simulink model "Standard"  (R2015a)
settings: Solver=ode45  StartTime=0.0  StopTime=300  RelTol=1e-3
undefined symbols (not defined in the file): A, B_cont, B_dist, dt, SegNum
settings Model: Creator=Nick  LastModifiedBy=Nick

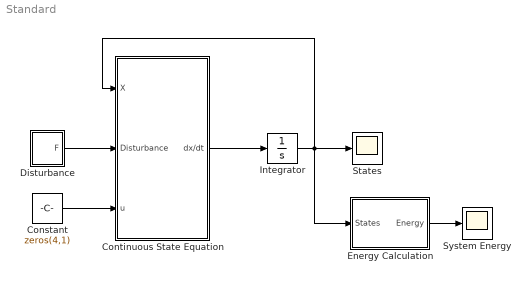
== system Standard ==
  Constant : Constant  Value=zeros(4,1)
  Continuous State Equation : Subsystem
  Disturbance : Subsystem
  Energy Calculation : Subsystem
  Integrator : Integrator
  States : Scope
      settings: SaveName=StandardStates
  System Energy : Scope
      settings: YMin=-5.65455e-27  YMax=3.5e-11  SaveName=StandardEnergy
  wires:
  Continuous State Equation/1(dx/dt) -> Integrator/1
  Integrator/1 -> States/1, Energy Calculation/1(States), Continuous State Equation/1(X)
  Energy Calculation/1(Energy) -> System Energy/1
  Disturbance/1(F) -> Continuous State Equation/2(Disturbance)
  Constant/1 -> Continuous State Equation/3(u)

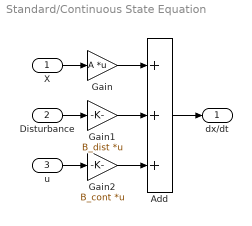
== system Standard/Continuous State Equation ==
  X : Inport
  Disturbance : Inport  Port=2
  u : Inport  Port=3
  Add : Sum  Inputs=+++
  Gain : Gain  Gain=A  Multiplication=Matrix(K*u)
  Gain1 : Gain  Gain=B_dist  Multiplication=Matrix(K*u)
  Gain2 : Gain  Gain=B_cont  Multiplication=Matrix(K*u)
  dx/dt : Outport
  wires:
  X/1 -> Gain/1
  Gain/1 -> Add/1
  Disturbance/1 -> Gain1/1
  Gain1/1 -> Add/2
  Add/1 -> dx/dt/1
  u/1 -> Gain2/1
  Gain2/1 -> Add/3

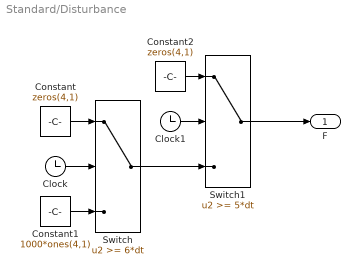
== system Standard/Disturbance ==
  Clock : Clock
  Clock1 : Clock
  Constant : Constant  Value=zeros(4,1)
  Constant1 : Constant  Value=1000*ones(4,1)
  Constant2 : Constant  Value=zeros(4,1)
  Switch : Switch  Threshold=6*dt
  Switch1 : Switch  Threshold=5*dt
  F : Outport
  wires:
  Clock/1 -> Switch/2
  Constant/1 -> Switch/1
  Constant1/1 -> Switch/3
  Switch/1 -> Switch1/3
  Constant2/1 -> Switch1/1
  Clock1/1 -> Switch1/2
  Switch1/1 -> F/1

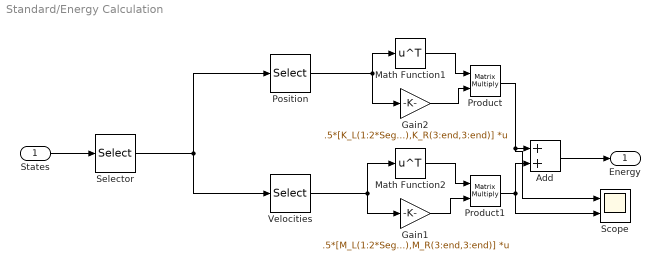
== system Standard/Energy Calculation ==
  States : Inport
  Add : Sum
  Gain1 : Gain  Gain=.5*[M_L(1:2*SegNum,1:2*SegNum),zeros(2*SegNum);zeros(2*SegNum),M_R(3:end,3:end)]  Multiplication=Matrix(K*u)
  Gain2 : Gain  Gain=.5*[K_L(1:2*SegNum,1:2*SegNum),zeros(2*SegNum);zeros(2*SegNum),K_R(3:end,3:end)]  Multiplication=Matrix(K*u)
  Math Function1 : Math  Operator=transpose  SaturateOnIntegerOverflow=on
  Math Function2 : Math  Operator=transpose  SaturateOnIntegerOverflow=on
  Position : Selector  InputPortWidth=length(A)-2  Indices=[1:SegNum*4]
  Product : Product  Multiplication=Matrix(*)  RndMeth=Zero
  Product1 : Product  Multiplication=Matrix(*)  RndMeth=Zero
  Scope : Scope  NumInputPorts=2
      settings: YMin=-5~-5  YMax=5~5
  Selector : Selector  InputPortWidth=length(A)  Indices=[1:2*SegNum,2*SegNum+2:6*SegNum+1,6*SegNum+3:length(A)]
  Velocities : Selector  InputPortWidth=length(A)-2  Indices=[SegNum*4+1:SegNum*8]
  Energy : Outport
  wires:
  Position/1 -> Gain2/1, Math Function1/1
  Math Function1/1 -> Product/1
  Gain2/1 -> Product/2
  Velocities/1 -> Gain1/1, Math Function2/1
  Math Function2/1 -> Product1/1
  Gain1/1 -> Product1/2
  Product/1 -> Scope/1, Add/1
  Product1/1 -> Scope/2, Add/2
  Add/1 -> Energy/1
  States/1 -> Selector/1
  Selector/1 -> Position/1, Velocities/1
